simulink model "linmodel_eq1_discr_2018a"  (R2018a)
settings: Solver=VariableStepAuto  StartTime=0.0  StopTime=30  RelTol=1e-3
InitFcn:
  | lin_discr_model
values from neighbouring files (symbols this model uses):
  A_eq1_d = sysd1.A    [MPC.m]    (also in MPC_sim.m)
  B_eq1_d = B_eq1_d(:,1)    [MPC.m]    (also in MPC_sim.m)
  C_eq1_d = sysd1.C    [MPC.m]    (also in MPC_sim.m)
  D_eq1_d = D_eq1_d(:,1)    [MPC.m]    (also in MPC_sim.m)
  Ts = 0.01    [MPC.m]    (also in MPC_main.m; MPC_new.m = 0.002; MPC_sim.m)
undefined symbols (not defined in the file or in its folder): A_L, B_L, C_L, D_L, Discrete, Time
libraries: ctrlSharedLib x1
settings Model: Creator=jessi  LastModifiedBy=jessi
settings DataIOCC: ReturnWorkspaceOutputs=on
settings SFSimCC: SimUseLocalCustomCode=on
settings RTWCC: RTWUseLocalCustomCode=on

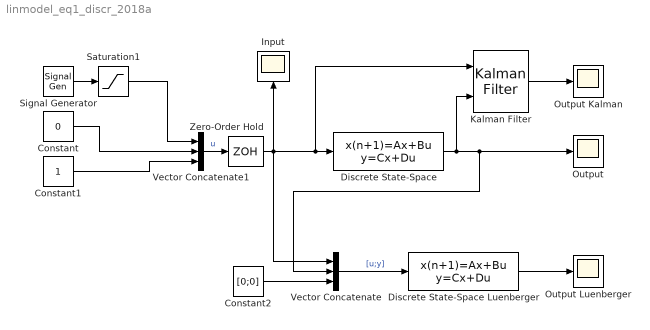
== system linmodel_eq1_discr_2018a ==
  Constant : Constant  Value=0
  Constant1 : Constant
  Constant2 : Constant  Value=[0;0]
  "Discrete State-Space " : DiscreteStateSpace  A=A_eq1_d  B=B_eq1_d  C=C_eq1_d  D=D_eq1_d  InitialCondition=[pi;0;0;0]  SampleTime=Ts
  Discrete State-Space Luenberger : DiscreteStateSpace  A=A_L  B=B_L  C=C_L  D=D_L  InitialCondition=[pi;0;0;0]  SampleTime=Ts
  Input : Scope
  Kalman Filter : ctrlSharedLib/Kalman Filter  TimeDomain=Discrete-Time  UseCurrentEstimator=on  ModelSource=Individual A, B, C, D matrices  ModelSourceVariable=ss(0.95,1,1,0,1)  A=A_eq1_d  B=B_eq1_d  C=C_eq1_d  D=D_eq1_d  NumberOfStates=1  NumberOfInputs=1  NumberOfOutputs=1  InitialEstimateSource=Dialog  X0=[pi;0;0;0]  P0=10  UseK=off  UseGH=off  NumberOfProcessNoiseInputs=1  G=1  TimeInvariantG=on  H=0  TimeInvariantH=on  Q=([0,0,0,0])  TimeInvariantQ=on  R=([0.0001,0.0001])  TimeInvariantR=on  N=0  TimeInvariantN=on  AddInputPort=on  AddEnablePort=off  OutputEstimatedY=off  OutputP=off  Ts=-1
      settings: SourceProductBaseCode=CT
  Output : Scope
  Output Kalman : Scope
  Output Luenberger : Scope
  Saturation1 : Saturate  UpperLimit=1  LowerLimit=-1
  Signal Generator : SignalGenerator  WaveForm=square  Amplitude=-0.3
  Vector Concatenate : Concatenate  NumInputs=3
  Vector Concatenate1 : Concatenate  NumInputs=3
  Zero-Order Hold : ZeroOrderHold  SampleTime=Ts
  wires:
  Constant/1 -> Vector Concatenate1/2
  Signal Generator/1 -> Saturation1/1
  Saturation1/1 -> Vector Concatenate1/1
  Constant1/1 -> Vector Concatenate1/3
  Vector Concatenate1/1 -> Zero-Order Hold/1  "u"
  Zero-Order Hold/1 -> Kalman Filter/1, "Discrete State-Space "/1, Vector Concatenate/1, Input/1
  "Discrete State-Space "/1 -> Kalman Filter/2, Vector Concatenate/2, Output/1
  Kalman Filter/1 -> Output Kalman/1
  Vector Concatenate/1 -> Discrete State-Space Luenberger/1  "[u;y]"
  Discrete State-Space Luenberger/1 -> Output Luenberger/1
  Constant2/1 -> Vector Concatenate/3
